simulink model "window_discriminator_5"  (R2018a)
settings: Solver=FixedStepAuto  StartTime=0.0  StopTime=6  RelTol=1e-3
PreLoadFcn:
  | load('alberto_data.mat')
model workspace (MAT data in the model file):
  dac_stop_max = 3
  threshold = [-50; -300]
  win_start = [0; 0]
  win_stop = [3; 3]
libraries: simulink x28, dspswit3 x2
settings Model: Creator=stefanobuccelli  LastModifiedBy=stefanobuccelli

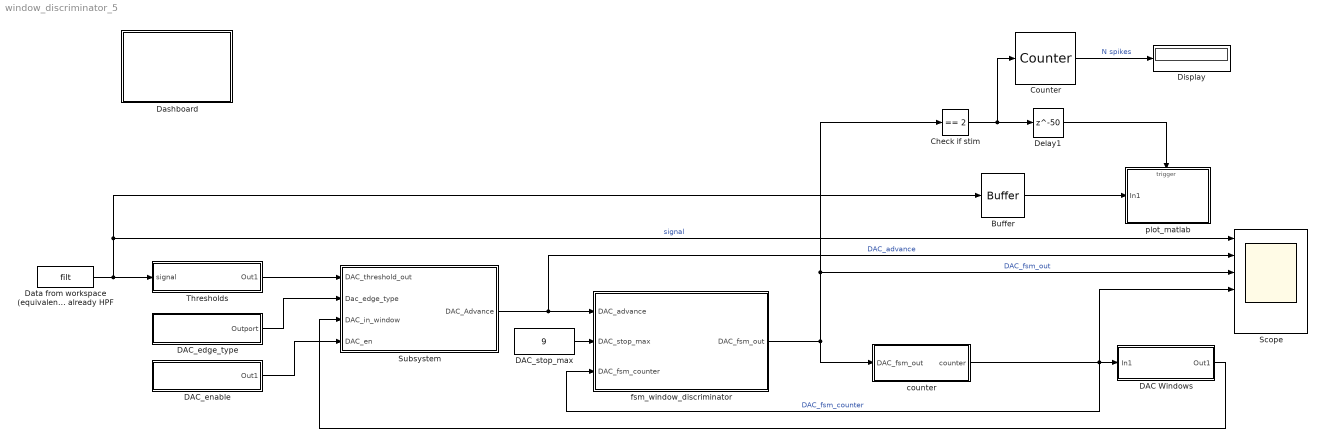
== system window_discriminator_5 ==
  Buffer : Buffer  N=100  V=99  OutputFrames=off
  Check if stim : simulink/Logic and Bit Operations/Compare To Constant  relop===  const=2  OutDataTypeStr=boolean
  Counter : dspswit3/Counter  Direction=Up  CountEvent=Rising edge  CounterSize=User defined  MaxCount=1e6  InitialCount=0  Output=Count  HitValue=32  ResetInput=off  SamplesPerFrame=1  Ts=1  CntDtype=double  HitDtype=Logical
  DAC Windows : Subsystem
  DAC_edge_type : Subsystem
  DAC_enable : Subsystem
  DAC_stop_max : Constant  Value=9  OutDataTypeStr=double
  Dashboard : Subsystem
  Data from workspace (equivalent to the board_DAC_data the one already HPF : FromWorkspace  VariableName=filt  SampleTime=1/25000
  Delay1 : Delay  DelayLength=50
  Display : Display
  Scope : Scope  NumInputPorts=6
  Subsystem : Subsystem
  Thresholds : Subsystem
  counter : Subsystem
  fsm_window_discriminator : Stateflow chart  TreatAsAtomicUnit=on
  plot_matlab : Subsystem
  wires:
  fsm_window_discriminator/1(DAC_fsm_out) -> counter/1(DAC_fsm_out), Check if stim/1, Scope/3  "DAC_fsm_out"
  Data from workspace (equivalent to the board_DAC_data the one already HPF/1 -> Buffer/1, Scope/1, Thresholds/1(signal)  "signal"
  Subsystem/1(DAC_Advance) -> Scope/2, fsm_window_discriminator/1(DAC_advance)  "DAC_advance"
  DAC_edge_type/1(Outport) -> Subsystem/2(Dac_edge_type)
  DAC_stop_max/1 -> fsm_window_discriminator/2(DAC_stop_max)
  Check if stim/1 -> Counter/1, Delay1/1
  Buffer/1 -> plot_matlab/1(In1)
  Delay1/1 -> plot_matlab/Trigger
  DAC Windows/1(Out1) -> Subsystem/3(DAC_in_window)
  Thresholds/1(Out1) -> Subsystem/1(DAC_threshold_out)
  DAC_enable/1(Out1) -> Subsystem/4(DAC_en)
  counter/1(counter) -> fsm_window_discriminator/3(DAC_fsm_counter), DAC Windows/1(In1), Scope/4  "DAC_fsm_counter"
  Counter/1 -> Display/1  "N spikes"

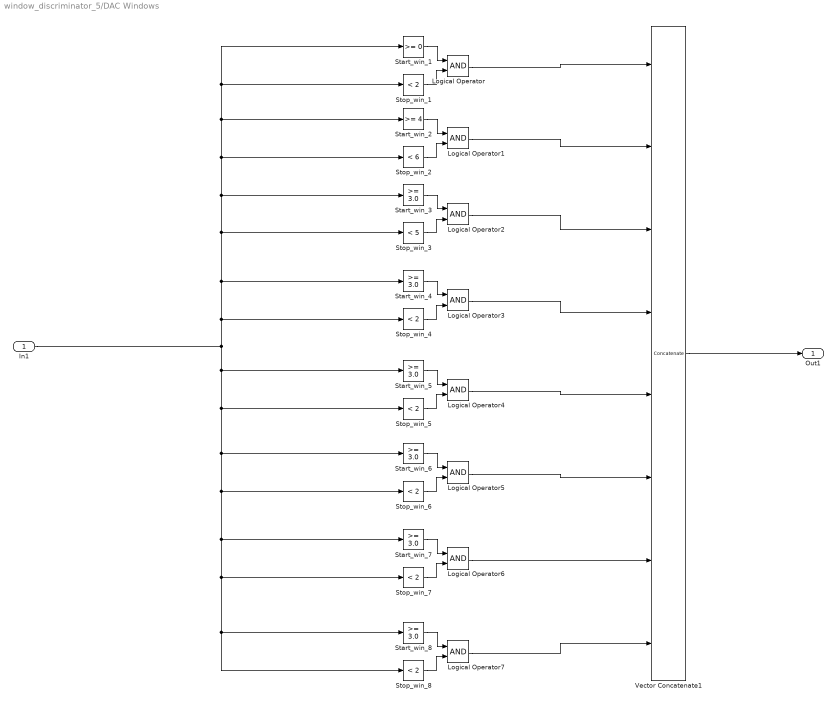
== system window_discriminator_5/DAC Windows ==
  In1 : Inport
  Logical Operator{,1..7} (8 alike) : Logic  AllPortsSameDT=off  OutDataTypeStr=boolean
  Start_win_1 : simulink/Logic and Bit Operations/Compare To Constant  relop=>=  const=0  OutDataTypeStr=boolean
  Start_win_2 : simulink/Logic and Bit Operations/Compare To Constant  relop=>=  const=4  OutDataTypeStr=boolean
  Start_win_{3..8} (6 alike) : simulink/Logic and Bit Operations/Compare To Constant  relop=>=  const=3.0  OutDataTypeStr=boolean
  Stop_win_{1,4..8} (6 alike) : simulink/Logic and Bit Operations/Compare To Constant  relop=<  const=2  OutDataTypeStr=boolean
  Stop_win_2 : simulink/Logic and Bit Operations/Compare To Constant  relop=<  const=6  OutDataTypeStr=boolean
  Stop_win_3 : simulink/Logic and Bit Operations/Compare To Constant  relop=<  const=5  OutDataTypeStr=boolean
  Vector Concatenate1 : Concatenate  NumInputs=8
  Out1 : Outport
  wires:
  Vector Concatenate1/1 -> Out1/1
  Stop_win_1/1 -> Logical Operator/2
  Start_win_1/1 -> Logical Operator/1
  Logical Operator/1 -> Vector Concatenate1/1
  Logical Operator1/1 -> Vector Concatenate1/2
  Stop_win_2/1 -> Logical Operator1/2
  Start_win_2/1 -> Logical Operator1/1
  Stop_win_3/1 -> Logical Operator2/2
  Start_win_3/1 -> Logical Operator2/1
  Logical Operator2/1 -> Vector Concatenate1/3
  Start_win_4/1 -> Logical Operator3/1
  Stop_win_4/1 -> Logical Operator3/2
  Logical Operator3/1 -> Vector Concatenate1/4
  Stop_win_5/1 -> Logical Operator4/2
  Start_win_5/1 -> Logical Operator4/1
  Logical Operator4/1 -> Vector Concatenate1/5
  Start_win_6/1 -> Logical Operator5/1
  Logical Operator5/1 -> Vector Concatenate1/6
  Stop_win_6/1 -> Logical Operator5/2
  Stop_win_7/1 -> Logical Operator6/2
  Start_win_7/1 -> Logical Operator6/1
  Logical Operator6/1 -> Vector Concatenate1/7
  Stop_win_8/1 -> Logical Operator7/2
  Start_win_8/1 -> Logical Operator7/1
  Logical Operator7/1 -> Vector Concatenate1/8
  In1/1 -> Stop_win_5/1, Start_win_6/1, Stop_win_6/1, Start_win_7/1, Stop_win_7/1, Start_win_8/1, Stop_win_8/1, Start_win_5/1, Stop_win_4/1, Start_win_4/1, Stop_win_3/1, Start_win_3/1, Stop_win_2/1, Start_win_2/1, Stop_win_1/1, Start_win_1/1

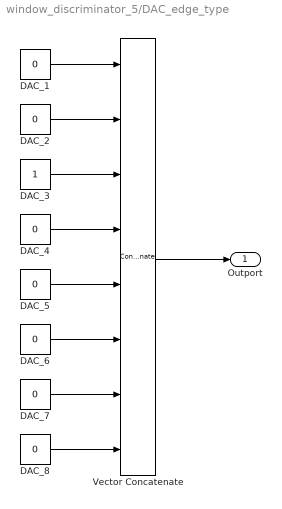
== system window_discriminator_5/DAC_edge_type ==
  DAC_{1..2,4..8} (7 alike) : Constant  Value=0
  DAC_3 : Constant
  Vector Concatenate : Concatenate  NumInputs=8
  Outport : Outport
  wires:
  DAC_7/1 -> Vector Concatenate/7
  DAC_6/1 -> Vector Concatenate/6
  DAC_1/1 -> Vector Concatenate/1
  Vector Concatenate/1 -> Outport/1
  DAC_5/1 -> Vector Concatenate/5
  DAC_8/1 -> Vector Concatenate/8
  DAC_4/1 -> Vector Concatenate/4
  DAC_3/1 -> Vector Concatenate/3
  DAC_2/1 -> Vector Concatenate/2

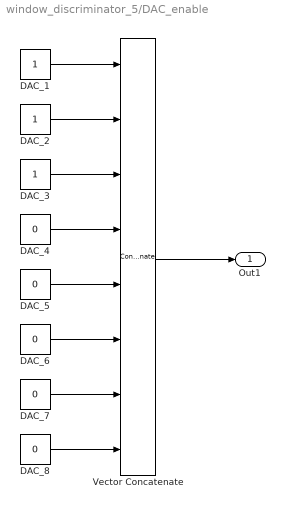
== system window_discriminator_5/DAC_enable ==
  DAC_1 : Constant
  DAC_2 : Constant
  DAC_3 : Constant
  DAC_{4..8} (5 alike) : Constant  Value=0
  Vector Concatenate : Concatenate  NumInputs=8
  Out1 : Outport
  wires:
  DAC_1/1 -> Vector Concatenate/1
  DAC_4/1 -> Vector Concatenate/4
  DAC_2/1 -> Vector Concatenate/2
  DAC_8/1 -> Vector Concatenate/8
  Vector Concatenate/1 -> Out1/1
  DAC_3/1 -> Vector Concatenate/3
  DAC_7/1 -> Vector Concatenate/7
  DAC_5/1 -> Vector Concatenate/5
  DAC_6/1 -> Vector Concatenate/6

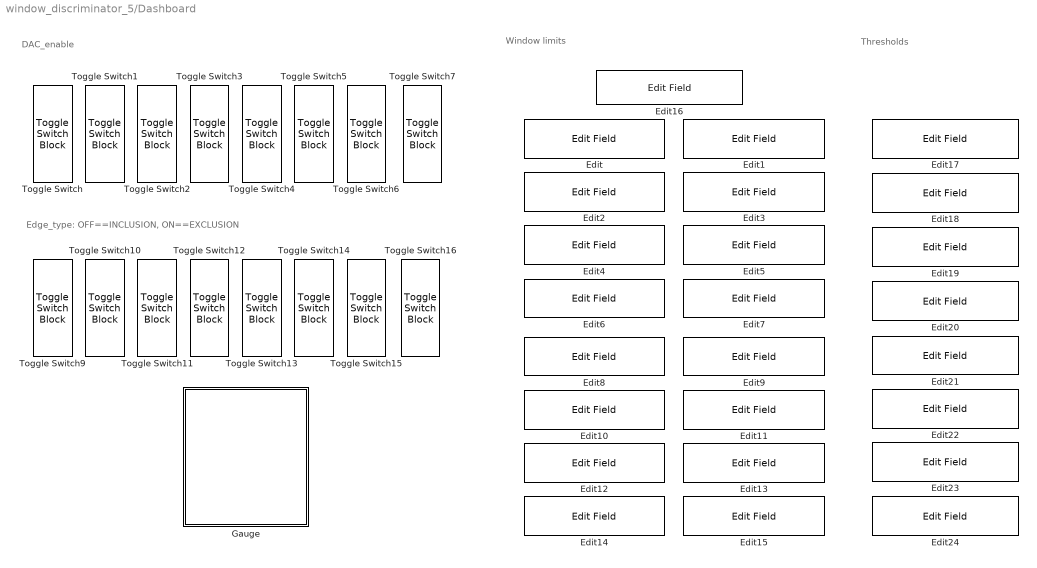
== system window_discriminator_5/Dashboard ==
  note: Thresholds
  note: Window limits
  note: Edge_type: OFF==INCLUSION, ON==EXCLUSION
  note: DAC_enable
  Edit : EditField  WebBlockId=147  Alignment=Center
  Edit1 : EditField  WebBlockId=149  Alignment=Center
  Edit10 : EditField  WebBlockId=158  Alignment=Center
  Edit11 : EditField  WebBlockId=159  Alignment=Center
  Edit12 : EditField  WebBlockId=160  Alignment=Center
  Edit13 : EditField  WebBlockId=161  Alignment=Center
  Edit14 : EditField  WebBlockId=162  Alignment=Center
  Edit15 : EditField  WebBlockId=163  Alignment=Center
  Edit16 : EditField  WebBlockId=243  Alignment=Center
  Edit17 : EditField  WebBlockId=264  Alignment=Center
  Edit18 : EditField  WebBlockId=257  Alignment=Center
  Edit19 : EditField  WebBlockId=258  Alignment=Center
  Edit2 : EditField  WebBlockId=150  Alignment=Center
  Edit20 : EditField  WebBlockId=259  Alignment=Center
  Edit21 : EditField  WebBlockId=260  Alignment=Center
  Edit22 : EditField  WebBlockId=261  Alignment=Center
  Edit23 : EditField  WebBlockId=262  Alignment=Center
  Edit24 : EditField  WebBlockId=263  Alignment=Center
  Edit3 : EditField  WebBlockId=151  Alignment=Center
  Edit4 : EditField  WebBlockId=152  Alignment=Center
  Edit5 : EditField  WebBlockId=153  Alignment=Center
  Edit6 : EditField  WebBlockId=154  Alignment=Center
  Edit7 : EditField  WebBlockId=155  Alignment=Center
  Edit8 : EditField  WebBlockId=156  Alignment=Center
  Edit9 : EditField  WebBlockId=157  Alignment=Center
  Gauge : Subsystem  DialogController=hmiCreateDDGDialog  IsWebBlock=on  mask(MWDashboardBlock){webBlockId=9508d0a0-9094-44a2-b73a-dcd38a83431a, webBlockType=circulargauge, ShowInLibBrowser=on, ShowInitialText=on, HMISrcModelName=window_discriminator_5}
      mask prompts: webBlockId "WebBlock Id"; webBlockType "WebBlock Type"; HMISrcModelName "Source Model"
      mask help: SimulinkHMI:dialogs:CircularGaugeDialogDesc
      mask Help: helpview([docroot '/mapfiles/simulink.map'], 'hmi_gauge')
      mask Display:
      | if strcmp(get_param(bdroot(gcb),'BlockDiagramType'), 'library')
      |     image([(matlabroot) '/toolbox/simulink/hmi/icons/CircularGauge.png']);
      | end
  Toggle Switch : ToggleSwitchBlock  WebBlockId=165
      settings: Values={{'Off', 'On'}, [0 1]}
  Toggle Switch1 : ToggleSwitchBlock  WebBlockId=177
      settings: Values={{'Off', 'On'}, [0 1]}
  Toggle Switch10 : ToggleSwitchBlock  WebBlockId=230
      settings: Values={{'Off', 'On'}, [0 1]}
  Toggle Switch11 : ToggleSwitchBlock  WebBlockId=231
      settings: Values={{'Off', 'On'}, [0 1]}
  Toggle Switch12 : ToggleSwitchBlock  WebBlockId=232
      settings: Values={{'Off', 'On'}, [0 1]}
  Toggle Switch13 : ToggleSwitchBlock  WebBlockId=233
      settings: Values={{'Off', 'On'}, [0 1]}
  Toggle Switch14 : ToggleSwitchBlock  WebBlockId=234
      settings: Values={{'Off', 'On'}, [0 1]}
  Toggle Switch15 : ToggleSwitchBlock  WebBlockId=235
      settings: Values={{'Off', 'On'}, [0 1]}
  Toggle Switch16 : ToggleSwitchBlock  WebBlockId=236
      settings: Values={{'Off', 'On'}, [0 1]}
  Toggle Switch2 : ToggleSwitchBlock  WebBlockId=181
      settings: Values={{'Off', 'On'}, [0 1]}
  Toggle Switch3 : ToggleSwitchBlock  WebBlockId=182
      settings: Values={{'Off', 'On'}, [0 1]}
  Toggle Switch4 : ToggleSwitchBlock  WebBlockId=183
      settings: Values={{'Off', 'On'}, [0 1]}
  Toggle Switch5 : ToggleSwitchBlock  WebBlockId=184
      settings: Values={{'Off', 'On'}, [0 1]}
  Toggle Switch6 : ToggleSwitchBlock  WebBlockId=185
      settings: Values={{'Off', 'On'}, [0 1]}
  Toggle Switch7 : ToggleSwitchBlock  WebBlockId=186
      settings: Values={{'Off', 'On'}, [0 1]}
  Toggle Switch9 : ToggleSwitchBlock  WebBlockId=229
      settings: Values={{'Off', 'On'}, [0 1]}

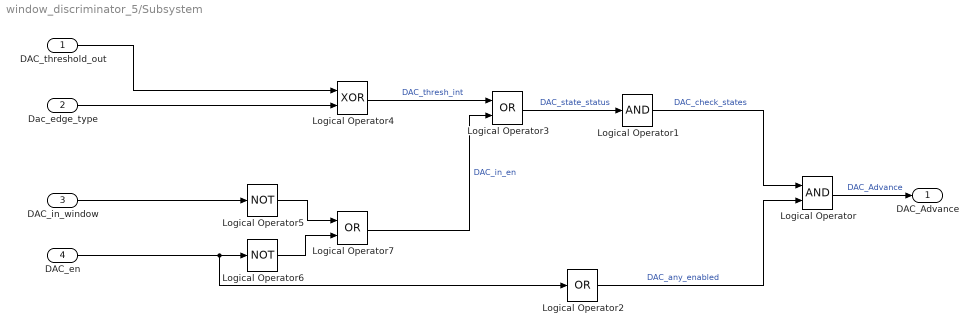
== system window_discriminator_5/Subsystem ==
  DAC_threshold_out : Inport
  Dac_edge_type : Inport  Port=2
  DAC_in_window : Inport  Port=3
  DAC_en : Inport  Port=4
  Logical Operator : Logic  AllPortsSameDT=off  OutDataTypeStr=boolean
  Logical Operator1 : Logic  Inputs=1  AllPortsSameDT=off  OutDataTypeStr=boolean
  Logical Operator2 : Logic  Operator=OR  Inputs=1  AllPortsSameDT=off  OutDataTypeStr=boolean
  Logical Operator3 : Logic  Operator=OR  AllPortsSameDT=off  OutDataTypeStr=boolean
  Logical Operator4 : Logic  Operator=XOR  AllPortsSameDT=off  OutDataTypeStr=boolean
  Logical Operator5 : Logic  Operator=NOT  Inputs=1  AllPortsSameDT=off  OutDataTypeStr=boolean
  Logical Operator6 : Logic  Operator=NOT  Inputs=1  AllPortsSameDT=off  OutDataTypeStr=boolean
  Logical Operator7 : Logic  Operator=OR  AllPortsSameDT=off  OutDataTypeStr=boolean
  DAC_Advance : Outport
  wires:
  Logical Operator/1 -> DAC_Advance/1  "DAC_Advance"
  Logical Operator2/1 -> Logical Operator/2  "DAC_any_enabled"
  Logical Operator1/1 -> Logical Operator/1  "DAC_check_states"
  Logical Operator4/1 -> Logical Operator3/1  "DAC_thresh_int"
  Logical Operator5/1 -> Logical Operator7/1
  DAC_threshold_out/1 -> Logical Operator4/1
  DAC_en/1 -> Logical Operator2/1, Logical Operator6/1
  Logical Operator3/1 -> Logical Operator1/1  "DAC_state_status"
  Logical Operator6/1 -> Logical Operator7/2
  Logical Operator7/1 -> Logical Operator3/2  "DAC_in_en"
  Dac_edge_type/1 -> Logical Operator4/2
  DAC_in_window/1 -> Logical Operator5/1

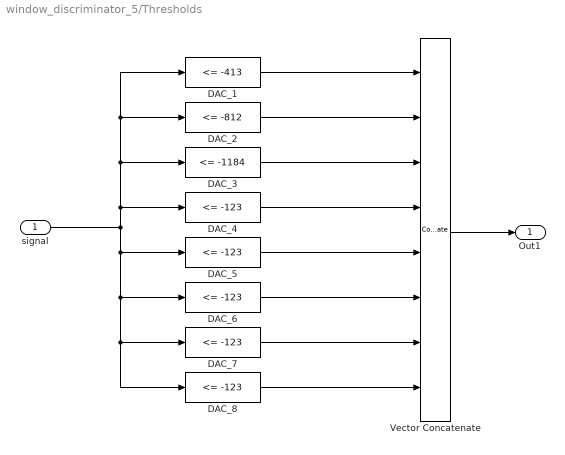
== system window_discriminator_5/Thresholds ==
  signal : Inport
  DAC_1 : simulink/Logic and Bit Operations/Compare To Constant  relop=<=  const=-413  OutDataTypeStr=boolean
  DAC_2 : simulink/Logic and Bit Operations/Compare To Constant  relop=<=  const=-812  OutDataTypeStr=boolean
  DAC_3 : simulink/Logic and Bit Operations/Compare To Constant  relop=<=  const=-1184  OutDataTypeStr=boolean
  DAC_{4..8} (5 alike) : simulink/Logic and Bit Operations/Compare To Constant  relop=<=  const=-123  OutDataTypeStr=boolean
  Vector Concatenate : Concatenate  NumInputs=8
  Out1 : Outport
  wires:
  Vector Concatenate/1 -> Out1/1
  signal/1 -> DAC_8/1, DAC_7/1, DAC_6/1, DAC_5/1, DAC_4/1, DAC_3/1, DAC_2/1, DAC_1/1
  DAC_1/1 -> Vector Concatenate/1
  DAC_2/1 -> Vector Concatenate/2
  DAC_4/1 -> Vector Concatenate/4
  DAC_3/1 -> Vector Concatenate/3
  DAC_6/1 -> Vector Concatenate/6
  DAC_7/1 -> Vector Concatenate/7
  DAC_5/1 -> Vector Concatenate/5
  DAC_8/1 -> Vector Concatenate/8

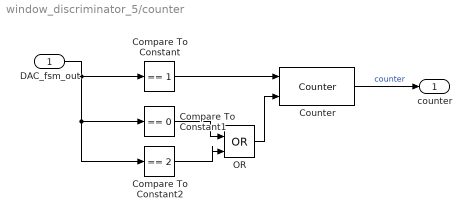
== system window_discriminator_5/counter ==
  DAC_fsm_out : Inport
  Compare To Constant : simulink/Logic and Bit Operations/Compare To Constant  relop===  const=1  OutDataTypeStr=boolean
  Compare To Constant1 : simulink/Logic and Bit Operations/Compare To Constant  relop===  const=0  OutDataTypeStr=boolean
  Compare To Constant2 : simulink/Logic and Bit Operations/Compare To Constant  relop===  const=2  OutDataTypeStr=boolean
  Counter : dspswit3/Counter  Direction=Up  CountEvent=Non-zero sample  CounterSize=User defined  MaxCount=255  InitialCount=0  Output=Count  HitValue=32  ResetInput=on  SamplesPerFrame=1  Ts=1  CntDtype=double  HitDtype=Logical
  OR : Logic  Operator=OR  IconShape=distinctive  AllPortsSameDT=off  OutDataTypeStr=boolean
  counter : Outport
  wires:
  Counter/1 -> counter/1  "counter"
  Compare To Constant2/1 -> OR/2
  Compare To Constant/1 -> Counter/1
  Compare To Constant1/1 -> OR/1
  OR/1 -> Counter/2
  DAC_fsm_out/1 -> Compare To Constant2/1, Compare To Constant1/1, Compare To Constant/1

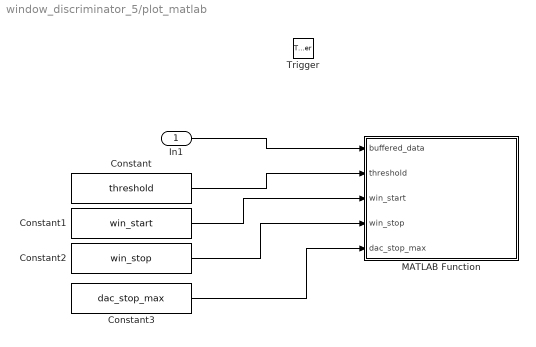
== system window_discriminator_5/plot_matlab ==
  In1 : Inport
  Trigger : TriggerPort  VariantControl=Variant  PortDimensions=1
  Constant : Constant  Value=threshold
  Constant1 : Constant  Value=win_start
  Constant2 : Constant  Value=win_stop
  Constant3 : Constant  Value=dac_stop_max
  MATLAB Function : MATLAB Function  TreatAsAtomicUnit=on
  wires:
  In1/1 -> MATLAB Function/1(buffered_data)
  Constant1/1 -> MATLAB Function/3(win_start)
  Constant/1 -> MATLAB Function/2(threshold)
  Constant2/1 -> MATLAB Function/4(win_stop)
  Constant3/1 -> MATLAB Function/5(dac_stop_max)

== system window_discriminator_5/Dashboard/Gauge ==

== matlab function window_discriminator_5/plot_matlab/MATLAB Function ==
  data: buffered_data input; threshold input; win_start input; win_stop input; dac_stop_max input
function  fcn(buffered_data,threshold,win_start,win_stop,dac_stop_max)
shift=length(buffered_data)/2;
figure(1)
plot((1:length(buffered_data))-shift,buffered_data,'k')
hold on
for curr_DAC=1:length(threshold)
    plot([win_start(curr_DAC):win_stop(curr_DAC)-1]-dac_stop_max,repmat(threshold(curr_DAC),1,length(win_start(curr_DAC):win_stop(curr_DAC)-1)),'b')
end
% the -1 in the start-stop win position is due to the delay (I guess XD)

== stateflow chart window_discriminator_5/fsm_window_discriminator ==
  settings: stateMachineType=MOORE_MACHINE  executeAtInitialization=1
  state IDLE
    DAC_fsm_out=0
  state TRACK
    DAC_fsm_out=1
  state STIM
    DAC_fsm_out=2
  (default) -> IDLE
  STIM -> IDLE
  TRACK -> IDLE [order 2] : [~DAC_advance]
  IDLE -> TRACK : [DAC_advance]
  TRACK -> TRACK [order 3] : [DAC_fsm_counter~=DAC_stop_max]
  TRACK -> STIM [order 1] : [DAC_fsm_counter==DAC_stop_max]
  data: DAC_advance input; DAC_fsm_out output double =0; DAC_stop_max input; DAC_fsm_counter input double =0
